simulink model "Grid_Forming_Converters_Microgrid_Github"  (R2020b)
settings: Solver=VariableStepAuto  StartTime=0.0  StopTime=1  RelTol=1e-3
values from neighbouring files (symbols this model uses):
  C_fi_1DG = 50*10^-6    (= 5e-05)    [Script_Primary_Secondary_Controller_GITHUB.m]
  C_fi_2DG = 50*10^-6    (= 5e-05)    [Script_Primary_Secondary_Controller_GITHUB.m]
  C_fi_3DG = 50*10^-6    (= 5e-05)    [Script_Primary_Secondary_Controller_GITHUB.m]
  C_fi_4DG = 50*10^-6    (= 5e-05)    [Script_Primary_Secondary_Controller_GITHUB.m]
  Kff_i_1DG = 0.75    [Script_Primary_Secondary_Controller_GITHUB.m]
  Kff_i_2DG = 0.75    [Script_Primary_Secondary_Controller_GITHUB.m]
  Kff_i_3DG = 0.75    [Script_Primary_Secondary_Controller_GITHUB.m]
  Kff_i_4DG = 0.75    [Script_Primary_Secondary_Controller_GITHUB.m]
  ki = 142500    [Script_Primary_Secondary_Controller_GITHUB.m]
  Kii_1DG = 20000    [Script_Primary_Secondary_Controller_GITHUB.m]
  Kii_2DG = 20000    [Script_Primary_Secondary_Controller_GITHUB.m]
  Kii_3DG = 16000    [Script_Primary_Secondary_Controller_GITHUB.m]
  Kii_4DG = 16000    [Script_Primary_Secondary_Controller_GITHUB.m]
  Kiv_1DG = 420    [Script_Primary_Secondary_Controller_GITHUB.m]
  Kiv_2DG = 420    [Script_Primary_Secondary_Controller_GITHUB.m]
  Kiv_3DG = 390    [Script_Primary_Secondary_Controller_GITHUB.m]
  Kiv_4DG = 390    [Script_Primary_Secondary_Controller_GITHUB.m]
  kp = 285    [Script_Primary_Secondary_Controller_GITHUB.m]
  Kpi_1DG = 15    [Script_Primary_Secondary_Controller_GITHUB.m]
  Kpi_2DG = 15    [Script_Primary_Secondary_Controller_GITHUB.m]
  Kpi_3DG = 10.5    [Script_Primary_Secondary_Controller_GITHUB.m]
  Kpi_4DG = 10.5    [Script_Primary_Secondary_Controller_GITHUB.m]
  Kpv_1DG = 0.1    [Script_Primary_Secondary_Controller_GITHUB.m]
  Kpv_2DG = 0.1    [Script_Primary_Secondary_Controller_GITHUB.m]
  Kpv_3DG = 0.05    [Script_Primary_Secondary_Controller_GITHUB.m]
  Kpv_4DG = 0.05    [Script_Primary_Secondary_Controller_GITHUB.m]
  L_ci_1DG = 0.35*10^-3    (= 0.00035)    [Script_Primary_Secondary_Controller_GITHUB.m]
  L_ci_2DG = 0.35*10^-3    (= 0.00035)    [Script_Primary_Secondary_Controller_GITHUB.m]
  L_fi_1DG = 1.35*10^-3    (= 0.00135)    [Script_Primary_Secondary_Controller_GITHUB.m]
  L_fi_2DG = 1.35*10^-3    (= 0.00135)    [Script_Primary_Secondary_Controller_GITHUB.m]
  L_fi_3DG = 1.35*10^-3    (= 0.00135)    [Script_Primary_Secondary_Controller_GITHUB.m]
  L_fi_4DG = 1.35*10^-3    (= 0.00135)    [Script_Primary_Secondary_Controller_GITHUB.m]
  L_line_1 = 318*10^-6    (= 0.000318)    [Script_Primary_Secondary_Controller_GITHUB.m]
  L_line_2 = 1847*10^-6    (= 0.001847)    [Script_Primary_Secondary_Controller_GITHUB.m]
  L_line_3 = 318*10^-6    (= 0.000318)    [Script_Primary_Secondary_Controller_GITHUB.m]
  L_load_1 = (X_load_1)/(2*pi*f)    (= 0.0477464829276)    [Script_Primary_Secondary_Controller_GITHUB.m]
  L_load_2 = (X_load_2)/(2*pi*f)    (= 0.0318309886184)    [Script_Primary_Secondary_Controller_GITHUB.m]
  L_load_3 = (X_load_3)/(2*pi*f)    (= 0.0318309886184)    [Script_Primary_Secondary_Controller_GITHUB.m]
  L_load_4 = (X_load_4)/(2*pi*f)    (= 0.0477464829276)    [Script_Primary_Secondary_Controller_GITHUB.m]
  m_P_1DG = 9.4*10^-5    (= 9.4e-05)    [Script_Primary_Secondary_Controller_GITHUB.m]
  m_P_2DG = 9.4*10^-5    (= 9.4e-05)    [Script_Primary_Secondary_Controller_GITHUB.m]
  m_P_3DG = 12.5*10^-5    (= 0.000125)    [Script_Primary_Secondary_Controller_GITHUB.m]
  m_P_4DG = 12.5*10^-5    (= 0.000125)    [Script_Primary_Secondary_Controller_GITHUB.m]
  n_Q_1DG = 1.3*10^-3    (= 0.0013)    [Script_Primary_Secondary_Controller_GITHUB.m]
  n_Q_2DG = 1.3*10^-3    (= 0.0013)    [Script_Primary_Secondary_Controller_GITHUB.m]
  n_Q_3DG = 1.5*10^-3    (= 0.0015)    [Script_Primary_Secondary_Controller_GITHUB.m]
  n_Q_4DG = 1.5*10^-3    (= 0.0015)    [Script_Primary_Secondary_Controller_GITHUB.m]
  R_ci_1DG = 0.03    [Script_Primary_Secondary_Controller_GITHUB.m]
  R_ci_2DG = 0.03    [Script_Primary_Secondary_Controller_GITHUB.m]
  R_fi_1DG = 0.1    [Script_Primary_Secondary_Controller_GITHUB.m]
  R_fi_2DG = 0.1    [Script_Primary_Secondary_Controller_GITHUB.m]
  R_fi_3DG = 0.1    [Script_Primary_Secondary_Controller_GITHUB.m]
  R_line_1 = 0.23    [Script_Primary_Secondary_Controller_GITHUB.m]
  R_line_2 = 0.35    [Script_Primary_Secondary_Controller_GITHUB.m]
  R_line_3 = 0.23    [Script_Primary_Secondary_Controller_GITHUB.m]
  R_load_1 = 30    [Script_Primary_Secondary_Controller_GITHUB.m]
  R_load_2 = 20    [Script_Primary_Secondary_Controller_GITHUB.m]
  R_load_3 = 25    [Script_Primary_Secondary_Controller_GITHUB.m]
  R_load_4 = 25    [Script_Primary_Secondary_Controller_GITHUB.m]
  Ts_1DG = 2e-6    (= 2e-06)    [Script_Primary_Secondary_Controller_GITHUB.m]
  w_base_1DG = 2*pi*f_1DG    (= 314.159265359)    [Script_Primary_Secondary_Controller_GITHUB.m]
  w_base_2DG = 2*pi*f_2DG    (= 314.159265359)    [Script_Primary_Secondary_Controller_GITHUB.m]
  w_base_3DG = 2*pi*f_3DG    (= 314.159265359)    [Script_Primary_Secondary_Controller_GITHUB.m]
  w_base_4DG = 2*pi*f_4DG    (= 314.159265359)    [Script_Primary_Secondary_Controller_GITHUB.m]
  wci_1DG = 31.41    [Script_Primary_Secondary_Controller_GITHUB.m]
  wci_2DG = 31.41    [Script_Primary_Secondary_Controller_GITHUB.m]
  wci_3DG = 31.41    [Script_Primary_Secondary_Controller_GITHUB.m]
  wci_4DG = 31.41    [Script_Primary_Secondary_Controller_GITHUB.m]
undefined symbols (not defined in the file or in its folder): L_i_1DG
libraries: powerlib x140, powerlib_meascontrol x68, pid_lib x20
(part 6 of 6)

== system Grid_Forming_Converters_Microgrid_Github/DG 4 VCVSI /Primary Controller DG 4/Voltage Loop Control 4 DG ==
  note: Is_d*
  note: Is_q*
  v_ref_dq0_4DG : Inport
  v_dq0_4DG : Inport  Port=2
  i_dq0_4DG : Inport  Port=3
  w_base_4DG : Inport  Port=4
  Demux : Demux  Outputs=2
  Demux1 : Demux  Outputs=2
  Demux2 : Demux  Outputs=2
  Gain : Gain  Gain=C_fi_4DG
  Gain1 : Gain  Gain=Kff_i_4DG
  Gain2 : Gain  Gain=Kff_i_4DG
  Is_0* : Constant  Value=0
  Mux : Mux  Inputs=3
  PID Controller : pid_lib/PID Controller  Controller=PI  Form=Parallel  TimeDomain=Continuous-time  UseExternalTs=off  SampleTime=-1  IntegratorMethod=Forward Euler  FilterMethod=Forward Euler  ControllerParametersSource=internal  P=Kpv_4DG  I=Kiv_4DG  D=0  UseFilter=on  N=100  TunerSelectOption=Transfer Function Based (PID Tuner App)  InitialConditionSource=internal  InitialConditionForIntegrator=0  InitialConditionForFilter=0  DifferentiatorICPrevScaledInput=0  ExternalReset=none  TrackingMode=off  Kt=1  LimitOutput=off  SatLimitsSource=internal  UpperSaturationLimit=inf  LowerSaturationLimit=-inf  LinearizeAsGain=on  AntiWindupMode=none  Kb=1  POutMin=[]  POutMax=[]  IOutMin=[]  IOutMax=[]  DOutMin=[]  DOutMax=[]  NOutMin=[]  NOutMax=[]  SumOutMin=[]  SumOutMax=[]  SaturationOutMin=[]  SaturationOutMax=[]  PParamMin=[]  PParamMax=[]  IParamMin=[]  IParamMax=[]  DParamMin=[]  DParamMax=[]  NParamMin=[]  NParamMax=[]  KbParamMin=[]  KbParamMax=[]  KtParamMin=[]  KtParamMax=[]  KbOutMin=[]  KbOutMax=[]  KtOutMin=[]  KtOutMax=[]  IntegratorOutMin=[]  IntegratorOutMax=[]  FilterOutMin=[]  FilterOutMax=[]  SumI1OutMin=[]  SumI1OutMax=[]  SumI2OutMin=[]  SumI2OutMax=[]  SumI3OutMin=[]  SumI3OutMax=[]  SumI4OutMin=[]  SumI4OutMax=[]  SumDOutMin=[]  SumDOutMax=[]  DifferentiatorOutMin=[]  DifferentiatorOutMax=[]  FilterDiffOutCoefMin=[]  FilterDiffOutCoefMax=[]  ReciprocalOutMin=[]  ReciprocalOutMax=[]  SumDenOutMin=[]  SumDenOutMax=[]  SumNumOutMin=[]  SumNumOutMax=[]  DivideOutMin=[]  DivideOutMax=[]  UdiffTsProdOutMin=[]  UdiffTsProdOutMax=[]  NTsProdOutMin=[]  NTsProdOutMax=[]  UintegralTsProdOutMin=[]  UintegralTsProdOutMax=[]  UngainTsProdOutMin=[]  UngainTsProdOutMax=[]  IntegratorContinuousStateAttributes=''  IntegratorStateMustResolveToSignalObject=off  IntegratorRTWStateStorageClass=Auto  FilterContinuousStateAttributes=''  FilterStateMustResolveToSignalObject=off  FilterRTWStateStorageClass=Auto  ParallelPVariant=InternalParameters  IdealPVariant=Disabled  IVariant=InternalParameters  DVariant=Disabled  IntegratorVariant=Continuous  SatVariant=Disabled  AWVariant=Passthrough  PCopyVariant=Disabled  TRVariant=Disabled  FdbkBlocksVariant=Forward  IdealPFdbkVariant=Disabled  SatFdbkVariant=Disabled  DerivativeFilterVariant=Disabled  NVariant=Disabled  NCopyVariant=Disabled_SignalSpec  FilterICVariant=Disabled  IntegratorICVariant=InternalICs  ExternalResetVariant=Disabled  TRSumVariant=Passthrough  SumFdbkVariant=Disabled  SumVariant=Sum_PI  TsampFilterVariant=InternalTs  TsampNgainVariant=Passthrough  TsampIntegralVariant=Passthrough  ExternalSaturationOutDataTypeStr=Inherit: Same as second input
  PID Controller2 : pid_lib/PID Controller  Controller=PI  Form=Parallel  TimeDomain=Continuous-time  UseExternalTs=off  SampleTime=-1  IntegratorMethod=Forward Euler  FilterMethod=Forward Euler  ControllerParametersSource=internal  P=Kpv_4DG  I=Kiv_4DG  D=0  UseFilter=on  N=100  TunerSelectOption=Transfer Function Based (PID Tuner App)  InitialConditionSource=internal  InitialConditionForIntegrator=0  InitialConditionForFilter=0  DifferentiatorICPrevScaledInput=0  ExternalReset=none  TrackingMode=off  Kt=1  LimitOutput=off  SatLimitsSource=internal  UpperSaturationLimit=inf  LowerSaturationLimit=-inf  LinearizeAsGain=on  AntiWindupMode=none  Kb=1  POutMin=[]  POutMax=[]  IOutMin=[]  IOutMax=[]  DOutMin=[]  DOutMax=[]  NOutMin=[]  NOutMax=[]  SumOutMin=[]  SumOutMax=[]  SaturationOutMin=[]  SaturationOutMax=[]  PParamMin=[]  PParamMax=[]  IParamMin=[]  IParamMax=[]  DParamMin=[]  DParamMax=[]  NParamMin=[]  NParamMax=[]  KbParamMin=[]  KbParamMax=[]  KtParamMin=[]  KtParamMax=[]  KbOutMin=[]  KbOutMax=[]  KtOutMin=[]  KtOutMax=[]  IntegratorOutMin=[]  IntegratorOutMax=[]  FilterOutMin=[]  FilterOutMax=[]  SumI1OutMin=[]  SumI1OutMax=[]  SumI2OutMin=[]  SumI2OutMax=[]  SumI3OutMin=[]  SumI3OutMax=[]  SumI4OutMin=[]  SumI4OutMax=[]  SumDOutMin=[]  SumDOutMax=[]  DifferentiatorOutMin=[]  DifferentiatorOutMax=[]  FilterDiffOutCoefMin=[]  FilterDiffOutCoefMax=[]  ReciprocalOutMin=[]  ReciprocalOutMax=[]  SumDenOutMin=[]  SumDenOutMax=[]  SumNumOutMin=[]  SumNumOutMax=[]  DivideOutMin=[]  DivideOutMax=[]  UdiffTsProdOutMin=[]  UdiffTsProdOutMax=[]  NTsProdOutMin=[]  NTsProdOutMax=[]  UintegralTsProdOutMin=[]  UintegralTsProdOutMax=[]  UngainTsProdOutMin=[]  UngainTsProdOutMax=[]  IntegratorContinuousStateAttributes=''  IntegratorStateMustResolveToSignalObject=off  IntegratorRTWStateStorageClass=Auto  FilterContinuousStateAttributes=''  FilterStateMustResolveToSignalObject=off  FilterRTWStateStorageClass=Auto  ParallelPVariant=InternalParameters  IdealPVariant=Disabled  IVariant=InternalParameters  DVariant=Disabled  IntegratorVariant=Continuous  SatVariant=Disabled  AWVariant=Passthrough  PCopyVariant=Disabled  TRVariant=Disabled  FdbkBlocksVariant=Forward  IdealPFdbkVariant=Disabled  SatFdbkVariant=Disabled  DerivativeFilterVariant=Disabled  NVariant=Disabled  NCopyVariant=Disabled_SignalSpec  FilterICVariant=Disabled  IntegratorICVariant=InternalICs  ExternalResetVariant=Disabled  TRSumVariant=Passthrough  SumFdbkVariant=Disabled  SumVariant=Sum_PI  TsampFilterVariant=InternalTs  TsampNgainVariant=Passthrough  TsampIntegralVariant=Passthrough  ExternalSaturationOutDataTypeStr=Inherit: Same as second input
  Product : Product
  Product1 : Product
  Scope1 : Scope
  Scope8 : Scope
  Selector1 : Selector  InputPortWidth=3  IndexOptions=Index vector (dialog)  Indices=[1 2]  OutputSizes=1
  Selector2 : Selector  InputPortWidth=3  IndexOptions=Index vector (dialog)  Indices=[1 2]  OutputSizes=1
  Selector3 : Selector  InputPortWidth=3  IndexOptions=Index vector (dialog)  Indices=[1 2]  OutputSizes=1
  Sum : Sum  Inputs=|+-
  Sum1 : Sum  Inputs=|+-
  Sum2 : Sum  Inputs=|+-
  Sum3 : Sum  Inputs=|++
  Sum4 : Sum  Inputs=|++
  Sum5 : Sum  Inputs=|++
  powergui : powerlib/powergui  Priority=1  SimulationMode=Discrete  SampleTime=2e-6  frequency=60  Iterations=50  frequencyindice=0  Pbase=100e6  ErrMax=1e-4  UnitsV=kV  UnitsW=MW  buscounter=0  FunctionMessages=off  echomessages=off  EnableUseOfTLC=off  CurrentSourceSwitches=off  DisableSnubberDevices=off  DisableRonSwitches=off  DisableVfSwitches=off  DisplayEquations=off  AutomaticDiscreteSolvers=off  SolverType=Tustin/Backward Euler (TBE)  Interpol=off  ExternalGateDelay=off  methode=off  Ts=100  x0status=blocks  SPID=on  SwTol=0  HookPort=off  NonlinearTolerance=1e-4  nMaxIteration=100  ContinueOnMaxIteration=off  RestoreLinks=warning  ResistiveCurrentMeasurement=off  Frange=[0:2:500]  Ylog=off  Xlog=on  ShowGrid=off  save=off  variable=ZData  structure=0  ZoomFFT=off  StartTime=0.0  cycles=1  DisplayStyle=1  fundamental=60  FreqAxis=off  MaxFrequency=1000  frequencyindicesteady=1  RmsSteady=1  display=off
  i_s_ref_dq0_4DG : Outport
  wires:
  v_ref_dq0_4DG/1 -> Selector1/1
  Selector1/1 -> Demux/1
  Demux/1 -> Sum/1  "Eg_d*"
  v_dq0_4DG/1 -> Selector2/1
  Selector2/1 -> Demux1/1
  Demux1/1 -> Scope8/1, Product1/1, Sum/2  "Eg_d"
  Demux/2 -> Sum1/1  "Eg_q*"
  Demux1/2 -> Sum1/2, Scope1/1, Product/2  "Eg_q"
  Sum1/1 -> PID Controller/1
  PID Controller/1 -> Sum3/1
  w_base_4DG/1 -> Gain/1
  Gain/1 -> Product1/2, Product/1
  Product/1 -> Sum2/2
  Sum2/1 -> Sum4/1
  i_dq0_4DG/1 -> Selector3/1
  Selector3/1 -> Demux2/1
  Product1/1 -> Sum3/2
  Sum3/1 -> Sum5/1
  Gain1/1 -> Sum4/2
  Demux2/1 -> Gain1/1  "Eg_d"
  Demux2/2 -> Gain2/1  "Eg_q"
  Gain2/1 -> Sum5/2
  Sum4/1 -> [i_1d_star_4DG], Mux/1
  Sum5/1 -> [i_1q_star_4DG], Mux/2
  Is_0*/1 -> Mux/3
  Mux/1 -> i_s_ref_dq0_4DG/1
  Sum/1 -> PID Controller2/1
  PID Controller2/1 -> Sum2/1

== system Grid_Forming_Converters_Microgrid_Github/DG 4 VCVSI /Primary Controller DG 4/convertion block dq to abc frame 4 DG ==
  v_s_ref_dq0_4DG : Inport
  alpha_4DG : Inport  Port=2
  Display23 : Display
  Scope48 : Scope
  dq0 to abc : powerlib_meascontrol/Transformations/dq0 to abc  Alignment=90 degrees behind phase A axis
  powergui : powerlib/powergui  Priority=1  SimulationMode=Discrete  SampleTime=2e-6  frequency=60  Iterations=50  frequencyindice=0  Pbase=100e6  ErrMax=1e-4  UnitsV=kV  UnitsW=MW  buscounter=0  FunctionMessages=off  echomessages=off  EnableUseOfTLC=off  CurrentSourceSwitches=off  DisableSnubberDevices=off  DisableRonSwitches=off  DisableVfSwitches=off  DisplayEquations=off  AutomaticDiscreteSolvers=off  SolverType=Tustin/Backward Euler (TBE)  Interpol=off  ExternalGateDelay=off  methode=off  Ts=100  x0status=blocks  SPID=on  SwTol=0  HookPort=off  NonlinearTolerance=1e-4  nMaxIteration=100  ContinueOnMaxIteration=off  RestoreLinks=warning  ResistiveCurrentMeasurement=off  Frange=[0:2:500]  Ylog=off  Xlog=on  ShowGrid=off  save=off  variable=ZData  structure=0  ZoomFFT=off  StartTime=0.0  cycles=1  DisplayStyle=1  fundamental=60  FreqAxis=off  MaxFrequency=1000  frequencyindicesteady=1  RmsSteady=1  display=off
  voltage_abc_DG4 : Outport
  wires:
  dq0 to abc/1 -> voltage_abc_DG4/1
  v_s_ref_dq0_4DG/1 -> Scope48/1, dq0 to abc/1, Display23/1
  alpha_4DG/1 -> dq0 to abc/2

== system Grid_Forming_Converters_Microgrid_Github/DG 1 VCVSI/Conversion and Measurement Block from abc to dq0 frame/Measurement block/Low Pass Filter d ==
  In1 : Inport
  Transfer Fcn1 : TransferFcn  Numerator=[wci_1DG]  Denominator=[1 wci_1DG]
  Out1 : Outport
  wires:
  In1/1 -> Transfer Fcn1/1
  Transfer Fcn1/1 -> Out1/1

== system Grid_Forming_Converters_Microgrid_Github/DG 1 VCVSI/Conversion and Measurement Block from abc to dq0 frame/Measurement block/Low Pass Filter q ==
  In1 : Inport
  Transfer Fcn1 : TransferFcn  Numerator=[wci_1DG]  Denominator=[1 wci_1DG]
  Out1 : Outport
  wires:
  In1/1 -> Transfer Fcn1/1
  Transfer Fcn1/1 -> Out1/1

== system Grid_Forming_Converters_Microgrid_Github/DG 2 VCVSI/Conversion and Measurement Block from abc to dq0 frame/Measurement block/Low Pass Filter d ==
  In1 : Inport
  Transfer Fcn1 : TransferFcn  Numerator=[wci_2DG]  Denominator=[1 wci_2DG]
  Out1 : Outport
  wires:
  In1/1 -> Transfer Fcn1/1
  Transfer Fcn1/1 -> Out1/1

== system Grid_Forming_Converters_Microgrid_Github/DG 2 VCVSI/Conversion and Measurement Block from abc to dq0 frame/Measurement block/Low Pass Filter q ==
  In1 : Inport
  Transfer Fcn1 : TransferFcn  Numerator=[wci_2DG]  Denominator=[1 wci_2DG]
  Out1 : Outport
  wires:
  In1/1 -> Transfer Fcn1/1
  Transfer Fcn1/1 -> Out1/1

== system Grid_Forming_Converters_Microgrid_Github/DG 3 VCVSI /Conversion and Measurement Block from abc to dq0 frame/Measurement block/Low Pass Filter d ==
  In1 : Inport
  Transfer Fcn1 : TransferFcn  Numerator=[wci_3DG]  Denominator=[1 wci_3DG]
  Out1 : Outport
  wires:
  In1/1 -> Transfer Fcn1/1
  Transfer Fcn1/1 -> Out1/1

== system Grid_Forming_Converters_Microgrid_Github/DG 3 VCVSI /Conversion and Measurement Block from abc to dq0 frame/Measurement block/Low Pass Filter q ==
  In1 : Inport
  Transfer Fcn1 : TransferFcn  Numerator=[wci_3DG]  Denominator=[1 wci_3DG]
  Out1 : Outport
  wires:
  In1/1 -> Transfer Fcn1/1
  Transfer Fcn1/1 -> Out1/1

== system Grid_Forming_Converters_Microgrid_Github/DG 4 VCVSI /Conversion and Measurement Block from abc to dq0 frame/Measurement block/Low Pass Filter d ==
  In1 : Inport
  Transfer Fcn1 : TransferFcn  Numerator=[wci_4DG]  Denominator=[1 wci_4DG]
  Out1 : Outport
  wires:
  In1/1 -> Transfer Fcn1/1
  Transfer Fcn1/1 -> Out1/1

== system Grid_Forming_Converters_Microgrid_Github/DG 4 VCVSI /Conversion and Measurement Block from abc to dq0 frame/Measurement block/Low Pass Filter q ==
  In1 : Inport
  Transfer Fcn1 : TransferFcn  Numerator=[wci_4DG]  Denominator=[1 wci_4DG]
  Out1 : Outport
  wires:
  In1/1 -> Transfer Fcn1/1
  Transfer Fcn1/1 -> Out1/1

== matlab function Grid_Forming_Converters_Microgrid_Github/DG 1 VCVSI/Secondary Controller DG 1 ==
  data: v_od_matrix input; P_matrix input; v_f_1DG output; Q_matrix input; w_matrix input; v_v_1DG output
function [v_f_1DG, v_v_1DG]  = SC_1DG(v_od_matrix, P_matrix, Q_matrix, w_matrix)

A_matrix= [0 0 0 0; 1 0 0 0; 0 1 0 0; 0 0 1 0]
g_pinning_gain= [1;0;0;0]
w_ref= 2*pi*50;
v_ref= 1;
c_f_1DG= 30;
c_v_1DG= 30;
m_P_1DG= 9.4*10^-5;
m_P_2DG= 9.4*10^-5;
m_P_3DG= 12.5*10^-5;
m_P_4DG= 12.5*10^-5;

n_Q_1DG= 1.3*10^-3;
n_Q_2DG= 1.3*10^-3; 
n_Q_3DG= 1.5*10^-3; 
n_Q_4DG= 1.5*10^-3; 

m_P_matrix= [m_P_1DG; m_P_2DG; m_P_3DG; m_P_4DG];
n_Q_matrix= [n_Q_1DG; n_Q_2DG; n_Q_3DG; n_Q_4DG];

%% Distributed frequency control for DG 1

x=0;

for i=1
    for j=1:4
        x= A_matrix(i,j)*(w_matrix(i) - w_matrix(j)) + x;
    end
    resul_1DG= g_pinning_gain(i)*(w_matrix(i) - w_ref);
end

x_1DG= resul_1DG + x;




y=0;

for i=1
    for j= 1:4
        y= A_matrix(i,j)*(m_P_matrix(i)*P_matrix(i) - m_P_matrix(j)*P_matrix(j)) + y;
    end
end

v_f_1DG= (-x_1DG - y)*(c_f_1DG);

%% Distributed voltage control for DG 1

z= 0;

for i= 1
    for j= 1:4
        z= A_matrix(i,j)*(v_od_matrix(i) - v_od_matrix(j)) + z;
    end
    result_1DG= g_pinning_gain(i)*(v_od_matrix(i) - v_ref)
end

z_1DG= result_1DG + z;

r= 0;

for i= 1
    for j= 1:4
        r= A_matrix(i,j)*(n_Q_matrix(i)*Q_matrix(i) - n_Q_matrix(j)*Q_matrix(j)) + r;
    end
end

v_v_1DG= (-z_1DG - r)*(c_v_1DG);

%% END

== matlab function Grid_Forming_Converters_Microgrid_Github/DG 4 VCVSI /Secondary Controller DG 4 ==
  data: v_od_matrix input; P_matrix input; v_f_4DG output; Q_matrix input; w_matrix input; v_v_4DG output
function [v_f_4DG, v_v_4DG]  = SC_4DG(v_od_matrix, P_matrix, Q_matrix, w_matrix)

A_matrix= [0 0 0 0; 1 0 0 0; 0 1 0 0; 0 0 1 0]
g_pinning_gain= [1;0;0;0]
w_ref= 2*pi*50;
v_ref= 1;
c_f_4DG= 30;
c_v_4DG= 30;
m_P_1DG= 9.4*10^-5;
m_P_2DG= 9.4*10^-5;
m_P_3DG= 12.5*10^-5;
m_P_4DG= 12.5*10^-5;
n_Q_1DG= 1.3*10^-3;
n_Q_2DG= 1.3*10^-3; 
n_Q_3DG= 1.5*10^-3; 
n_Q_4DG= 1.5*10^-3; 

m_P_matrix= [m_P_1DG; m_P_2DG; m_P_3DG; m_P_4DG];
n_Q_matrix= [n_Q_1DG; n_Q_2DG; n_Q_3DG; n_Q_4DG];

%% Distributed frequency control for DG 4

x=0;

for i=4
    for j=1:4
        x= A_matrix(i,j)*(w_matrix(i) - w_matrix(j)) + x;
    end
    resul_4DG= g_pinning_gain(i)*(w_matrix(i) - w_ref);
end

x_4DG= resul_4DG + x;




y=0;

for i=4
    for j= 1:4
        y= A_matrix(i,j)*(m_P_matrix(i)*P_matrix(i) - m_P_matrix(j)*P_matrix(j)) + y;
    end
end

v_f_4DG= (-x_4DG - y)*(c_f_4DG);

%% Distributed voltage control for DG 4

z= 0;

for i= 4
    for j= 1:4
        z= A_matrix(i,j)*(v_od_matrix(i) - v_od_matrix(j)) + z;
    end
    result_4DG= g_pinning_gain(i)*(v_od_matrix(i) - v_ref);
end

z_4DG= result_4DG + z;

r= 0;

for i= 4
    for j= 1:4
        r= A_matrix(i,j)*(n_Q_matrix(i)*Q_matrix(i) - n_Q_matrix(j)*Q_matrix(j)) + r;
    end
end

v_v_4DG= (-z_4DG - r)*(c_v_4DG);

%% END

== matlab function Grid_Forming_Converters_Microgrid_Github/DG 2 VCVSI/Secondary Controller DG 2 VCVSI ==
  data: v_od_matrix input; P_matrix input; v_f_2DG output; Q_matrix input; w_matrix input; v_v_2DG output
function [v_f_2DG, v_v_2DG]  = SC_2DG(v_od_matrix, P_matrix, Q_matrix, w_matrix)

A_matrix= [0 0 0 0; 1 0 0 0; 0 1 0 0; 0 0 1 0]
g_pinning_gain= [1;0;0;0]
w_ref= 2*pi*50;
v_ref= 1;
c_f_2DG= 30;
c_v_2DG= 30;
m_P_1DG= 9.4*10^-5;
m_P_2DG= 9.4*10^-5;
m_P_3DG= 12.5*10^-5;
m_P_4DG= 12.5*10^-5;

n_Q_1DG= 1.3*10^-3;
n_Q_2DG= 1.3*10^-3; 
n_Q_3DG= 1.5*10^-3; 
n_Q_4DG= 1.5*10^-3; 



m_P_matrix= [m_P_1DG; m_P_2DG; m_P_3DG; m_P_4DG];
n_Q_matrix= [n_Q_1DG; n_Q_2DG; n_Q_3DG; n_Q_4DG];

%% Distributed frequency control for DG 2

x=0;

for i=2
    for j=1:4
        x= A_matrix(i,j)*(w_matrix(i) - w_matrix(j)) + x;
    end
    resul_2DG= g_pinning_gain(i)*(w_matrix(i) - w_ref);
end

x_2DG= resul_2DG + x;




y=0;

for i=2
    for j= 1:4
        y= A_matrix(i,j)*(m_P_matrix(i)*P_matrix(i) - m_P_matrix(j)*P_matrix(j)) + y;
    end
end

v_f_2DG= (-x_2DG - y)*(c_f_2DG);

%% Distributed voltage control for DG 2

z= 0;

for i= 2
    for j= 1:4
        z= A_matrix(i,j)*(v_od_matrix(i) - v_od_matrix(j)) + z;
    end
    result_2DG= g_pinning_gain(i)*(v_od_matrix(i) - v_ref);
end

z_2DG= result_2DG + z;

r= 0;

for i= 2
    for j= 1:4
        r= A_matrix(i,j)*(n_Q_matrix(i)*Q_matrix(i) - n_Q_matrix(j)*Q_matrix(j)) + r;
    end
end

v_v_2DG= (-z_2DG - r)*(c_v_2DG);

%% END

== matlab function Grid_Forming_Converters_Microgrid_Github/DG 3 VCVSI /Secondary Controller DG 3 VCVSI ==
  data: v_od_matrix input; P_matrix input; v_f_3DG output; Q_matrix input; w_matrix input; v_v_3DG output
function [v_f_3DG, v_v_3DG]  = SC_3DG(v_od_matrix, P_matrix, Q_matrix, w_matrix)

A_matrix= [0 0 0 0; 1 0 0 0; 0 1 0 0; 0 0 1 0];
g_pinning_gain= [1;0;0;0];
w_ref= 2*pi*50;
v_ref= 1;
c_f_3DG= 30;
c_v_3DG= 30;
m_P_1DG= 9.4*10^-5;
m_P_2DG= 9.4*10^-5;
m_P_3DG= 12.5*10^-5;
m_P_4DG= 12.5*10^-5;

n_Q_1DG= 1.3*10^-3;
n_Q_2DG= 1.3*10^-3; 
n_Q_3DG= 1.5*10^-3; 
n_Q_4DG= 1.5*10^-3; 

m_P_matrix= [m_P_1DG; m_P_2DG; m_P_3DG; m_P_4DG];
n_Q_matrix= [n_Q_1DG; n_Q_2DG; n_Q_3DG; n_Q_4DG];

%% Distributed frequency control for DG 3

x=0;

for i=3
    for j=1:4
        x= A_matrix(i,j)*(w_matrix(i) - w_matrix(j)) + x;
    end
    resul_3DG= g_pinning_gain(i)*(w_matrix(i) - w_ref);
end

x_3DG= resul_3DG + x;




y=0;

for i=3
    for j= 1:4
        y= A_matrix(i,j)*(m_P_matrix(i)*P_matrix(i) - m_P_matrix(j)*P_matrix(j)) + y;
    end
end

v_f_3DG= (-x_3DG - y)*(c_f_3DG);

%% Distributed voltage control for DG 3

z= 0;

for i= 3
    for j= 1:4
        z= A_matrix(i,j)*(v_od_matrix(i) - v_od_matrix(j)) + z;
    end
    result_3DG= g_pinning_gain(i)*(v_od_matrix(i) - v_ref);
end

z_3DG= result_3DG + z;

r= 0;

for i= 3
    for j= 1:4
        r= A_matrix(i,j)*(n_Q_matrix(i)*Q_matrix(i) - n_Q_matrix(j)*Q_matrix(j)) + r;
    end
end

v_v_3DG= (-z_3DG - r)*(c_v_3DG);

%% END
